simulink model "symmetric_lht"  (R2020a)
settings: Solver=FixedStepDiscrete  StartTime=0.0  StopTime=inf  RelTol=1e-3
values from neighbouring files (symbols this model uses):
  fs = fclk(1)*1e6    [setupSystem.m]
  height = heightName(nameIdx)    [setupSystem.m]
  inarray = uint8(simDirNew)    [setupSystem.m]
  nRho = maxRho*2    [setupSystem.m]
  nTheta = length(theta)    [setupSystem.m]
  theta = 0:1:179    [SymmetricLHT.m]    (also in setupSystem.m = (0:1:179))
  width = widthName(nameIdx)    [setupSystem.m]
undefined symbols (not defined in the file or in its folder): rhoBits, rhoMax
libraries: hdlsllib x35, simulink x25, dspsrcs4 x1
(part 2 of 2)

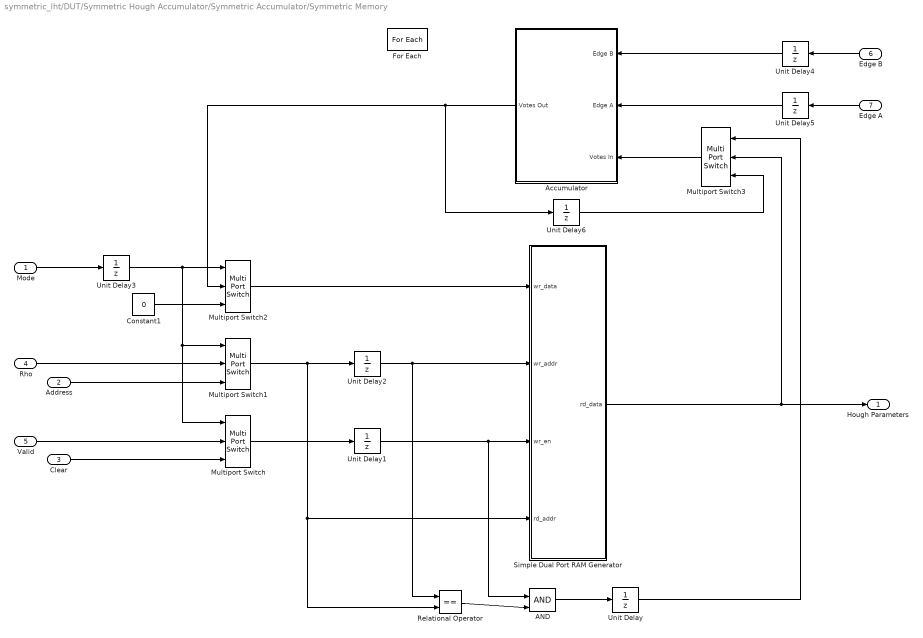
== system symmetric_lht/DUT/Symmetric Hough Accumulator/Symmetric Accumulator/Symmetric Memory ==
  Mode : Inport
  Address : Inport  Port=2
  Clear : Inport  Port=3
  Rho : Inport  Port=4  Partition=on  PartitionDimension=2  PartitionWidth=1  PartitionOffset=0
  Valid : Inport  Port=5
  Edge B : Inport  Port=6
  Edge A : Inport  Port=7
  AND : Logic  IconShape=distinctive  AllPortsSameDT=off  OutDataTypeStr=boolean
  Accumulator : Subsystem
  Constant1 : Constant  Value=0  OutDataTypeStr=fixdt(0,rhoBits*2,0)  SampleTime=-1
  For Each : ForEach  DisableCoverage=on
  Multiport Switch{,1..3} (4 alike) : MultiPortSwitch  DataPortOrder=Zero-based contiguous  Inputs=2  zeroidx=on
  Relational Operator : RelationalOperator  Operator===  OutDataTypeStr=boolean  RndMeth=Simplest
  Simple Dual Port RAM Generator : Subsystem  VariantControl=other_bits  mask{b=22, d=1470, b_hidden=22, d_hidden=1470}
      mask prompts: b "Data width:"; d "Depth:"
      mask init:
      | if d == d_hidden
      |     return
      | end
      | 
      | dBase = evalin('base', get_param(gcb, 'd'));
      | bBase = evalin('base', get_param(gcb, 'b'));
      | 
      | fprintf('HPS Memory updated...\r\n');
      | 
      | set_param(gcb, 'd_hidden', int2str(dBase));
      | set_param(gcb, 'b_hidden', int2str(bBase));
      | 
      | % Xilinx RAM Initialisation
      | xl_config = [512, 72;
      |             1024, 36;
      |             2048, 18;
      |             4096, 9;
      |             8192, 4;
      |             16384, 2;
      |             32768, 1];
      | 
      | % Get length of Xilinx Configuration
      | sizeram = size(xl_config);
      |         
      | % Get the RAM Configuration based on the data width
      | for i = 1:sizeram(1)
      |     if b <= xl_config(i, 2)
      |         a = xl_config(i, :);
      |     end
      | end
      | 
      | % Get number of BRAM required (including half BRAM)
      | numbram = ceil((d/a(1))/0.5)*0.5;
      | fullbram = floor(numbram); % Integer
      | halfbram = (numbram-floor(numbram)) ~= 0; % Boolean
      | 
      | % Get all blocks and delete everything excepts ports
      | H = get(find_system(gcb, 'FindAll', 'on', 'type', 'block'));
      | todelete = setdiff(strcat(repmat({[gcb '/']}, numel(H.Blocks), 1),  H.Blocks),...
      |     strcat(repmat({[gcb '/']}, 5, 1),...
      |     {'wr_data'; 'wr_addr'; 'wr_en'; 'rd_addr'; 'rd_data'}));
      | delete_block(todelete);
      | 
      | % Delete lines
      | for i = 1:numel(H.Lines)
      |     delete_line(H.Lines(i).Handle)
      | end
      | 
      | % Generate full BRAMs
      | y = 0;
      | 
      | % If there is only one ram then the write enable should be directly
      | % connected to the first ram write enable. Else, the write address must be sliced
      | % and the upper bound (over a(2)) compared to zero. This will indicate if
      | % the first ram is the one to be written/read from.
      | 
      | % Common to both implementations
      | % Write Address Slice
      | add_block('hdlsllib/Logic and Bit Operations/Bit Slice',...
      |         [gcb, '/wr_address'], 'Position',...
      |         [160 130 250 170]);
      | % Set bitslice parameters
      | set_param([gcb, '/wr_address'],...
      |     'lidx', int2str(log2(a(1))-1));
      | set_param([gcb, '/wr_address'],...
      |     'ridx', int2str(0));
      | 
      | % Read Address Slice
      | add_block('hdlsllib/Logic and Bit Operations/Bit Slice',...
      |         [gcb, '/rd_address'], 'Position',...
      |         [160 330 250 370]);
      | % Set bitslice parameters
      | set_param([gcb, '/rd_address'],...
      |     'lidx', int2str(log2(a(1))-1));
      | set_param([gcb, '/rd_address'],...
      |     'ridx', int2str(0));
      | 
      | if ceil(numbram) == 1
      |     
      |     i = 1;
      |     
      |     % Set bitslice parameters
      |     set_param([gcb, '/rd_address'],...
      |         'lidx', int2str(ceil(log2(d))-1));
      |     set_param([gcb, '/wr_address'],...
      |         'lidx', int2str(ceil(log2(d))-1));
      |     
      |     % Add Simple RAM
      |     add_block('hdlsllib/HDL RAMs/Simple Dual Port RAM',...
      |         [gcb, '/simple_ram_', int2str(i-1)], 'Position',...
      |         [635 0+600*y 635+200 400+600*y]);
      | 
      |     % Set RAM parameters
      |     set_param([gcb, '/simple_ram_', int2str(i-1)],...
      |         'ram_size', int2str(ceil(log2(d))));
      | 
      |     % Connect "wr_data" to "simple_ram_i"
      |     add_line(gcb, ['wr_data/1'], ['simple_ram_', int2str(i-1), '/1'],...
      |         'autorouting', 'on');
      |     
      |     % Connect "wr_addr" to "wr_address"
      |     add_line(gcb, ['wr_addr/1'], ['wr_address/1'],...
      |         'autorouting', 'on');
      | 
      |     % Connect "wr_address" to "simple_ram_i"
      |     add_line(gcb, ['wr_address/1'], ['simple_ram_', int2str(i-1), '/2'],...
      |         'autorouting', 'on');
      | 
      |     % Connect "wr_en" to "simple_ram_i"
      |     add_line(gcb, ['wr_en/1'], ['simple_ram_', int2str(i-1), '/3'],...
      |         'autorouting', 'on');
      |     
      |     % Connect "rd_addr" to "rd_address"
      |     add_line(gcb, ['rd_addr/1'], ['rd_address/1'],...
      |         'autorouting', 'on');
      | 
      |     % Connect "rd_address" to "simple_ram_i"
      |     add_line(gcb, ['rd_address/1'], ['simple_ram_', int2str(i-1), '/4'],...
      |         'autorouting', 'on');
      |     
      |     % Connect "simple_ram_i" to "rd_data"
      |     add_line(gcb, ['simple_ram_', int2str(i-1), '/1'], ['rd_data/1'],...
      |         'autorouting', 'on');
      | 
      | else
      |     
      |     % Multiport Switch
      |     add_block('hdlsllib/Signal Routing/Multiport Switch',...
      |         [gcb, '/multiport_switch'], 'Position',...
      |         [1340 146 1405 250]);
      |     % Set multiport switch parameters
      |     set_param([gcb, '/multiport_switch'],...
      |         'Inputs', int2str(ceil(numbram)));
      |     set_param([gcb, '/multiport_switch'],...
      |         'DataPortOrder', 'Zero-based contiguous');
      | 
      |     % Add Constant Zero
      |     add_block('hdlsllib/Sources/Constant',...
      |         [gcb, '/zero'], 'Position',...
      |         [425 -65 455 -35]);
      |     set_param([gcb, '/zero'],...
      |         'Value', int2str(0));
      |     set_param([gcb, '/zero'],...
      |         'OutDataTypeStr', ['fixdt(0, ', int2str(ceil(numbram)), ', 0)']);
      | 
      |     % Add Vector Concatenate
      |     add_block('hdlsllib/Signal Routing/Vector Concatenate',...
      |         [gcb, '/vector_concatenate'], 'Position',...
      |         [1015, -113, 1025, 38]);
      |     set_param([gcb, '/vector_concatenate'],...
      |         'NumInputs', int2str(ceil(numbram)));
      | 
      |     % Add Bitwise-OR
      |     add_block('hdlsllib/Logic and Bit Operations/Bitwise Operator',...
      |         [gcb, '/bitwise_or'], 'Position',...
      |         [1165, -54, 1205, -16]);
      |     set_param([gcb, '/bitwise_or'],...
      |         'logicop', 'OR');
      |     set_param([gcb, '/bitwise_or'],...
      |         'UseBitMask', 0);
      |     set_param([gcb, '/bitwise_or'],...
      |         'NumInputPorts', int2str(1));
      | 
      |     % Add delay for bram access
      |     add_block('hdlsllib/Discrete/Delay',...
      |         [gcb, '/delay'], 'Position',...
      |         [1248, 60, 1282, 95]);
      |     set_param([gcb, '/delay'],...
      |         'DelayLength', int2str(1));
      |     
      |     % Add bitslice
      |     add_block('hdlsllib/Logic and Bit Operations/Bit Slice',...
      |         [gcb, '/wr_bitslice'], 'Position',...
      |         [-65 180 25 220]);
      | 
      |     % Set bitslice parameters
      |     set_param([gcb, '/wr_bitslice'],...
      |         'lidx', int2str(ceil(log2(d)-1)));
      |     set_param([gcb, '/wr_bitslice'],...
      |         'ridx', int2str(log2(a(1))));
      |     
      |     % Add bitslice
      |     add_block('hdlsllib/Logic and Bit Operations/Bit Slice',...
      |         [gcb, '/rd_bitslice'], 'Position',...
      |         [-65 280 25 320]);
      | 
      |     % Set bitslice parameters
      |     set_param([gcb, '/rd_bitslice'],...
      |         'lidx', int2str(ceil(log2(d)-1)));
      |     set_param([gcb, '/rd_bitslice'],...
      |         'ridx', int2str(log2(a(1))));
      |     
      |     for i = 1:ceil(numbram)
      |         
      |         %%%%% Begin Adding Blocks %%%%%
      |         % Add Simple RAM
      |         add_block('hdlsllib/HDL RAMs/Simple Dual Port RAM',...
      |             [gcb, '/simple_ram_', int2str(i-1)], 'Position',...
      |             [635 0+600*y 635+200 400+600*y]);
      | 
      |         % Set RAM parameters
      |         set_param([gcb, '/simple_ram_', int2str(i-1)],...
      |             'ram_size', int2str(log2(a(1))));
      | 
      |         % Add compare to constant
      |         add_block('hdlsllib/Logic and Bit Operations/Compare To Constant',...
      |             [gcb, '/wr_cmp2const_', int2str(i-1)], 'Position',...
      |             [190 225+y*600 220 255+y*600]); 
      | 
      |         % Set compare to zero parameters
      |         set_param([gcb, '/wr_cmp2const_', int2str(i-1)],...
      |             'relop', '==');
      | 
      |         % Set compare to zero parameters
      |         set_param([gcb, '/wr_cmp2const_', int2str(i-1)],...
      |             'const', int2str(i-1));
      |         
      |         % Add compare to constant
      |         add_block('hdlsllib/Logic and Bit Operations/Compare To Constant',...
      |             [gcb, '/rd_cmp2const_', int2str(i-1)], 'Position',...
      |             [190 445+y*600 220 475+y*600]); 
      | 
      |         % Set compare to zero parameters
      |         set_param([gcb, '/rd_cmp2const_', int2str(i-1)],...
      |             'relop', '==');
      | 
      |         % Set compare to zero parameters
      |         set_param([gcb, '/rd_cmp2const_', int2str(i-1)],...
      |             'const', int2str(i-1));
      | 
      |         % Add and logic
      |         add_block('hdlsllib/Logic and Bit Operations/Logical Operator',...
      |             [gcb, '/and_', int2str(i-1)], 'Position',...
      |             [420 231+600*y 455 264+600*y]);
      | 
      |         % Set and logic parameters
      |         set_param([gcb, '/and_', int2str(i-1)],...
      |             'Operator', 'AND');
      | 
      |         % Add Switch
      |         add_block('hdlsllib/Signal Routing/Switch',...
      |             [gcb, '/switch_', int2str(i-1)], 'Position',...
      |             [685 -113+600*y 785 -37+600*y]);
      | 
      |         % Set switch parameters
      |         set_param([gcb, '/switch_', int2str(i-1)],...
      |             'Threshold', int2str(1));
      | 
      |         % Add Constant
      |         add_block('hdlsllib/Sources/Constant',...
      |             [gcb, '/constant_', int2str(i-1)], 'Position',...
      |             [425 -115+600*y 455 -85+600*y]);
      | 
      |         % Set Constant parameters
      |         set_param([gcb, '/constant_', int2str(i-1)],...
      |             'Value', int2str(i-1));
      |         set_param([gcb, '/constant_', int2str(i-1)],...
      |             'OutDataTypeStr', ['fixdt(0, ', int2str(ceil(numbram)), ', 0)']);   
      | 
      |         %%%%% Begin Wire Connections %%%%%        
      |         % Connect "wr_data" to "simple_ram_i"
      |         add_line(gcb, 'wr_data/1', ['simple_ram_', int2str(i-1), '/1'],...
      |             'autorouting','on');
      | 
      |         % Connect "wr_address" to "simple_ram_i"
      |         add_line(gcb, 'wr_address/1', ['simple_ram_', int2str(i-1), '/2'],...
      |             'autorouting','on');
      | 
      |         % Connect "rd_address" to "simple_ram_i"
      |         add_line(gcb, 'rd_address/1', ['simple_ram_', int2str(i-1), '/4'],...
      |             'autorouting','on');
      | 
      |         % Connect "constant_i" to "switch_i"
      |         add_line(gcb, ['constant_', int2str(i-1), '/1'], ['switch_', int2str(i-1), '/1'],...
      |             'autorouting','on');
      | 
      |         % Connect "zero" to "switch_i"
      |         add_line(gcb, 'zero/1', ['switch_', int2str(i-1), '/3'],...
      |             'autorouting','on');
      | 
      |         % Connect "switch_i" to "vector_concatenate"
      |         add_line(gcb, ['switch_', int2str(i-1), '/1'], ['vector_concatenate/', int2str(i)],...
      |             'autorouting','on');
      | 
      |         % Connect "rd_address" to "simple_ram_i"
      |         add_line(gcb, ['simple_ram_', int2str(i-1), '/1'], ['multiport_switch/', int2str(i+1)],...
      |             'autorouting','on');
      | 
      |         % Connect "bitslice_i" to "wr_cmp2const_i"
      |         add_line(gcb, ['wr_bitslice/1'], ['wr_cmp2const_', int2str(i-1), '/1'],...
      |             'autorouting','on');
      |         
      |         % Connect "bitslice_i" to "rd_cmp2const_i"
      |         add_line(gcb, ['rd_bitslice/1'], ['rd_cmp2const_', int2str(i-1), '/1'],...
      |             'autorouting','on');
      | 
      |         % Connect "wr_en" to "and_i"
      |         add_line(gcb, ['wr_en/1'], ['and_', int2str(i-1), '/2'],...
      |             'autorouting','on');
      | 
      |         % Connect "and_i" to "simple_ram_0"
      |         add_line(gcb, ['and_', int2str(i-1), '/1'], ['simple_ram_', int2str(i-1), '/3'],...
      |             'autorouting','on');
      | 
      |         % Connect "wr_cmp2const_i" to "and_i"
      |         add_line(gcb, ['wr_cmp2const_', int2str(i-1), '/1'], ['and_', int2str(i-1), '/1'],...
      |             'autorouting','on');
      | 
      |         % Connect "rd_cmp2const_i" to "switch_i"
      |         add_line(gcb, ['rd_cmp2const_', int2str(i-1), '/1'], ['switch_', int2str(i-1), '/2'],...
      |             'autorouting','on');
      |          
      |         % Update coordinates
      |         y = y + 1;
      |         
      |     end
      |     
      |     % Connect "rd_addr" to "bitslice_i"
      |     add_line(gcb, ['rd_addr/1'], ['rd_bitslice/1'],...
      |         'autorouting','on');
      |     
      |     % Connect "wr_addr" to "bitslice_i"
      |     add_line(gcb, ['wr_addr/1'], ['wr_bitslice/1'],...
      |         'autorouting','on');
      |     
      |     % Connect "wr_addr" to "wr_address"
      |     add_line(gcb, 'wr_addr/1', ['wr_address', '/1'],...
      |         'autorouting','on');
      | 
      |     % Connect "rd_addr" to "rd_address"
      |     add_line(gcb, 'rd_addr/1', ['rd_address', '/1'],...
      |         'autorouting','on');
      | 
      |     % Connect "vector_concatenate" to "bitwise_or"
      |     add_line(gcb, ['vector_concatenate/1'], ['bitwise_or/1'],...
      |         'autorouting','on');
      | 
      |     % Connect "bitwise_or" to "delay"
      |     add_line(gcb, ['bitwise_or/1'], ['delay/1'],...
      |         'autorouting','on');
      | 
      |     % Connect "delay" to "multiport_switch"
      |     add_line(gcb, ['delay/1'], ['multiport_switch/1'],...
      |         'autorouting','on');
      | 
      |     % Connect "multiport_switch" to "rd_data"
      |     add_line(gcb, ['multiport_switch/1'], ['rd_data/1'],...
      |         'autorouting','on');
      |     
      | end
      | 
      | % If there is a half bram we must change a few parameters. Firstly, delete
      | % the write and read address lines. Then add bitslice blocks to reduce the
      | % address space in half. Connect rd_addr and wr_addr to the corresponding ports
      | % on the bram. Finally, change the address depth.
      | if halfbram
      |     
      |     if ceil(numbram) > 1
      |         
      |         % Delete lines
      |         delete_line(gcb, ['wr_address/1'], ['simple_ram_', int2str(i-1), '/2'])
      |         delete_line(gcb, ['rd_address/1'], ['simple_ram_', int2str(i-1), '/4'])
      |         
      |         % Write Address half ram Slice
      |         add_block('hdlsllib/Logic and Bit Operations/Bit Slice',...
      |                 [gcb, '/wr_address_hr'], 'Position',...
      |                 [160 130+(y-1)*600 250 170+(y-1)*600]);
      |         % Set bitslice parameters
      |         set_param([gcb, '/wr_address_hr'],...
      |             'lidx', int2str(log2(a(1))-2));
      |         set_param([gcb, '/wr_address_hr'],...
      |             'ridx', int2str(0));
      | 
      |         % Read Address half ram Slice
      |         add_block('hdlsllib/Logic and Bit Operations/Bit Slice',...
      |                 [gcb, '/rd_address_hr'], 'Position',...
      |                 [160 330+(y-1)*600 250 370+(y-1)*600]);
      |         % Set bitslice parameters
      |         set_param([gcb, '/rd_address_hr'],...
      |             'lidx', int2str(log2(a(1))-2));
      |         set_param([gcb, '/rd_address_hr'],...
      |             'ridx', int2str(0));
      | 
      |         % Connect "wr_addr" to "wr_address_hr"
      |         add_line(gcb, 'wr_addr/1', ['wr_address_hr', '/1'],...
      |             'autorouting','on');
      | 
      |         % Connect "rd_addr" to "rd_address_hr"
      |         add_line(gcb, 'rd_addr/1', ['rd_address_hr', '/1'],...
      |             'autorouting','on');
      | 
      |         % Connect "wr_address_hr" to "simple_ram_i"
      |         add_line(gcb, ['wr_address_hr', '/1'], ['simple_ram_', int2str(i-1), '/2'],...
      |             'autorouting','on');
      | 
      |         % Connect "rd_address_hr" to "simple_ram_i"
      |         add_line(gcb, ['rd_address_hr', '/1'], ['simple_ram_', int2str(i-1), '/4'],...
      |             'autorouting','on');
      |         
      |         % Update the ram parameters (address bits)
      |         set_param([gcb, '/simple_ram_', int2str(i-1)],...
      |             'ram_size', int2str(log2(a(1)/2)));
      | 
      |     else
      |         % Set bitslice parameters
      |         % set_param([gcb, '/wr_address'],...
      |         %     'lidx', int2str(log2(a(1))-2));
      |         % set_param([gcb, '/wr_address'],...
      |         %     'ridx', int2str(0));
      |         % Set bitslice parameters
      |         % set_param([gcb, '/rd_address'],...
      |         %     'lidx', int2str(log2(a(1))-2));
      |         % set_param([gcb, '/rd_address'],...
      |         %     'ridx', int2str(0));
      |         
      |     end
      |     
      | 
      |     
      | end
  Unit Delay{,1..6} (7 alike) : UnitDelay  SampleTime=-1  HasFrameUpgradeWarning=on
  Hough Parameters : Outport  ConcatenationDimension=2
  wires:
  Unit Delay/1 -> Multiport Switch3/1
  Unit Delay6/1 -> Multiport Switch3/3
  Multiport Switch3/1 -> Accumulator/3(Votes In)
  AND/1 -> Unit Delay/1
  Relational Operator/1 -> AND/2
  Valid/1 -> Multiport Switch/2
  Simple Dual Port RAM Generator/1(rd_data) -> Multiport Switch3/2, Hough Parameters/1
  Unit Delay5/1 -> Accumulator/2(Edge A)
  Unit Delay4/1 -> Accumulator/1(Edge B)
  Constant1/1 -> Multiport Switch2/3
  Unit Delay2/1 -> Simple Dual Port RAM Generator/2(wr_addr), Relational Operator/1
  Unit Delay1/1 -> Simple Dual Port RAM Generator/3(wr_en), AND/1
  Rho/1 -> Multiport Switch1/2
  Clear/1 -> Multiport Switch/3
  Unit Delay3/1 -> Multiport Switch/1, Multiport Switch1/1, Multiport Switch2/1
  Multiport Switch2/1 -> Simple Dual Port RAM Generator/1(wr_data)
  Multiport Switch/1 -> Unit Delay1/1
  Mode/1 -> Unit Delay3/1
  Edge B/1 -> Unit Delay4/1
  Address/1 -> Multiport Switch1/3
  Edge A/1 -> Unit Delay5/1
  Multiport Switch1/1 -> Simple Dual Port RAM Generator/4(rd_addr), Relational Operator/2, Unit Delay2/1
  Accumulator/1(Votes Out) -> Multiport Switch2/2, Unit Delay6/1

== system symmetric_lht/DUT/Symmetric Hough Kernel/FIFO Half Rate System/FIFO Half Rate A ==
  In : Inport
  Push : Inport  Port=2
  Delay : Delay  DelayLength=1
  HDL FIFO : hdlsllib/HDL RAMs/HDL FIFO  fifo_size=(width/2)/2+1  mode=Classic  ratio=2  push_msg=Error  pop_msg=Error  show_empty=on  show_full=off  show_num=off  LabelModeActiveChoice_Mode=Classic
      settings: SourceProductBaseCode=SL
  NOT : Logic  Operator=NOT  IconShape=distinctive  AllPortsSameDT=off  OutDataTypeStr=boolean
  Rate Transition : RateTransition
  Out : Outport
  Valid : Outport  Port=2
  wires:
  HDL FIFO/2 -> Rate Transition/1
  Push/1 -> HDL FIFO/2
  In/1 -> HDL FIFO/1
  HDL FIFO/1 -> Out/1
  Rate Transition/1 -> NOT/1
  NOT/1 -> HDL FIFO/3, Delay/1
  Delay/1 -> Valid/1

== system symmetric_lht/DUT/Symmetric Hough Kernel/FIFO Half Rate System/FIFO Half Rate B ==
  In : Inport
  Push : Inport  Port=2
  Delay : Delay  DelayLength=1
  HDL FIFO : hdlsllib/HDL RAMs/HDL FIFO  fifo_size=(width/2)/2+1  mode=Classic  ratio=2  push_msg=Error  pop_msg=Error  show_empty=on  show_full=off  show_num=off  LabelModeActiveChoice_Mode=Classic
      settings: SourceProductBaseCode=SL
  NOT : Logic  Operator=NOT  IconShape=distinctive  AllPortsSameDT=off  OutDataTypeStr=boolean
  Rate Transition : RateTransition
  Out : Outport
  Valid : Outport  Port=2
  wires:
  Delay/1 -> Valid/1
  NOT/1 -> Delay/1, HDL FIFO/3
  Rate Transition/1 -> NOT/1
  HDL FIFO/1 -> Out/1
  In/1 -> HDL FIFO/1
  Push/1 -> HDL FIFO/2
  HDL FIFO/2 -> Rate Transition/1

== system symmetric_lht/DUT/Symmetric Hough Kernel/Symmetric Kernel/Coordinate Counters ==
  valid : Inport
  AND : Logic  IconShape=distinctive  AllPortsSameDT=off  OutDataTypeStr=boolean
  Compare To Constant : simulink/Logic and Bit Operations/Compare To Constant  relop===  const=width/2  OutDataTypeStr=boolean
  Compare To Zero : simulink/Logic and Bit Operations/Compare To Zero  relop=>=  OutDataTypeStr=boolean
  Compare To Zero1 : simulink/Logic and Bit Operations/Compare To Zero  relop=>=  OutDataTypeStr=boolean
  Counter : hdlsllib/Sources/HDL Counter  CountType=Count limited  CountInit=-height/2  CountStep=1  CountMax=height/2-1  CountFromType=Initial value  CountFrom=-height/2  CountResetPort=off  CountLoadPort=off  CountEnbPort=on  CountDirPort=off  CountDataType=Signed  CountWordLen=ceil(log2(height+1))  CountFracLen=0  CountSampTime=1
  Increment Real World : simulink/Additional Math & Discrete/Additional Math: Increment - Decrement/Increment Real World
      settings: SourceProductBaseCode=SL
  Increment Real World1 : simulink/Additional Math & Discrete/Additional Math: Increment - Decrement/Increment Real World
      settings: SourceProductBaseCode=SL
  Multiport Switch : MultiPortSwitch  DataPortOrder=Zero-based contiguous  Inputs=2  zeroidx=on
  Multiport Switch1 : MultiPortSwitch  DataPortOrder=Zero-based contiguous  Inputs=2  zeroidx=on
  X Counter : hdlsllib/Sources/HDL Counter  CountType=Count limited  CountInit=1  CountStep=1  CountMax=width/2  CountFromType=Initial value  CountFrom=1  CountResetPort=off  CountLoadPort=off  CountEnbPort=on  CountDirPort=off  CountDataType=Unsigned  CountWordLen=ceil(log2(width/2+1))  CountFracLen=0  CountSampTime=1
  x : Outport  VectorParamsAs1DForOutWhenUnconnected=off
  y : Outport  Port=2  VectorParamsAs1DForOutWhenUnconnected=off
  yp1 : Outport  Port=3  VectorParamsAs1DForOutWhenUnconnected=off
  y relative : Outport  Port=4  VectorParamsAs1DForOutWhenUnconnected=off
  wires:
  valid/1 -> AND/2, X Counter/1
  X Counter/1 -> x/1, Compare To Constant/1
  AND/1 -> Counter/1
  Compare To Constant/1 -> AND/1
  Multiport Switch/1 -> y/1
  Counter/1 -> Multiport Switch/2, y relative/1, Increment Real World/1, Compare To Zero/1
  Compare To Zero/1 -> Multiport Switch/1
  Increment Real World1/1 -> Multiport Switch1/3
  Compare To Zero1/1 -> Multiport Switch1/1
  Increment Real World/1 -> Increment Real World1/1, Multiport Switch1/2, Compare To Zero1/1, Multiport Switch/3
  Multiport Switch1/1 -> yp1/1

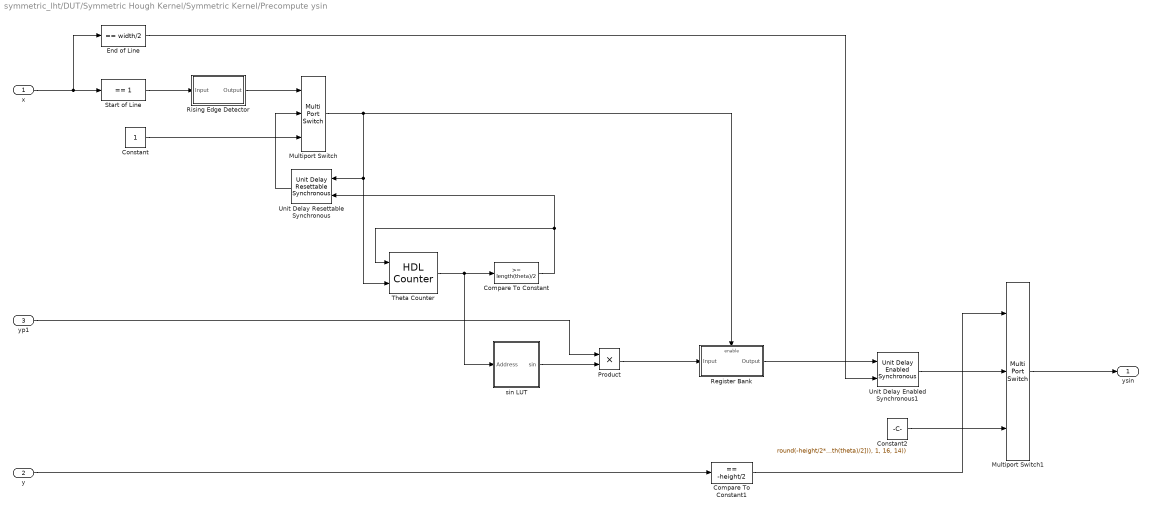
== system symmetric_lht/DUT/Symmetric Hough Kernel/Symmetric Kernel/Precompute ysin ==
  x : Inport
  y : Inport  Port=2
  yp1 : Inport  Port=3
  Compare To Constant : simulink/Logic and Bit Operations/Compare To Constant  relop=>=  const=length(theta)/2  OutDataTypeStr=boolean
  Compare To Constant1 : simulink/Logic and Bit Operations/Compare To Constant  relop===  const=-height/2  OutDataTypeStr=boolean
  Constant : Constant  OutDataTypeStr=boolean  SampleTime=-1
  Constant2 : Constant  Value=round(-height/2*fi(sin(deg2rad([0:1:length(theta)/2])), 1, 16, 14))  OutDataTypeStr=fixdt(1,ceil(log2(height+1)),0)  SampleTime=-1
  End of Line : simulink/Logic and Bit Operations/Compare To Constant  relop===  const=width/2  OutDataTypeStr=boolean
  Multiport Switch : MultiPortSwitch  DataPortOrder=Zero-based contiguous  Inputs=2  zeroidx=on
  Multiport Switch1 : MultiPortSwitch  DataPortOrder=Zero-based contiguous  Inputs=2  zeroidx=on
  Product : Product  RndMeth=Round  SaturateOnIntegerOverflow=on  OutDataTypeStr=Inherit: Same as first input
  Register Bank : Subsystem
  Rising Edge Detector : Subsystem
  Start of Line : simulink/Logic and Bit Operations/Compare To Constant  relop===  const=1  OutDataTypeStr=boolean
  Theta Counter : hdlsllib/Sources/HDL Counter  CountType=Count limited  CountInit=0  CountStep=1  CountMax=length(theta)/2  CountFromType=Initial value  CountFrom=0  CountResetPort=on  CountLoadPort=off  CountEnbPort=on  CountDirPort=off  CountDataType=Unsigned  CountWordLen=ceil(log2(length(theta)))  CountFracLen=0  CountSampTime=1
  Unit Delay Enabled Synchronous1 : hdlsllib/Discrete/Unit Delay Enabled Synchronous  InitialCondition=0.0  SampleTime=-1
      settings: SourceProductBaseCode=SL
  Unit Delay Resettable Synchronous : hdlsllib/Discrete/Unit Delay Resettable Synchronous  InitialCondition=0.0  SampleTime=-1
      settings: SourceProductBaseCode=SL
  sin LUT : Subsystem
  ysin : Outport  VectorParamsAs1DForOutWhenUnconnected=off
  wires:
  x/1 -> End of Line/1, Start of Line/1
  Start of Line/1 -> Rising Edge Detector/1(Input)
  Multiport Switch/1 -> Register Bank/Enable, Unit Delay Resettable Synchronous/1, Theta Counter/2
  Unit Delay Resettable Synchronous/1 -> Multiport Switch/2
  Constant/1 -> Multiport Switch/3
  Theta Counter/1 -> sin LUT/1(Address), Compare To Constant/1
  Rising Edge Detector/1(Output) -> Multiport Switch/1
  Multiport Switch1/1 -> ysin/1
  Constant2/1 -> Multiport Switch1/3
  Compare To Constant1/1 -> Multiport Switch1/1
  Product/1 -> Register Bank/1(Input)
  y/1 -> Compare To Constant1/1
  Compare To Constant/1 -> Unit Delay Resettable Synchronous/2, Theta Counter/1
  Unit Delay Enabled Synchronous1/1 -> Multiport Switch1/2
  End of Line/1 -> Unit Delay Enabled Synchronous1/2
  Register Bank/1(Output) -> Unit Delay Enabled Synchronous1/1
  yp1/1 -> Product/1
  sin LUT/1(sin) -> Product/2

== system symmetric_lht/DUT/Symmetric Hough Kernel/Symmetric Kernel/Quadrant Control ==
  Valid : Inport
  Delay : Delay  DelayLength=1  ShowEnablePort=on
      settings: InputPortMap=u0,e6
  First Quadrant Valid : Logic  IconShape=distinctive  AllPortsSameDT=off  OutDataTypeStr=boolean
  NOT : Logic  Operator=NOT  IconShape=distinctive  AllPortsSameDT=off  OutDataTypeStr=boolean
  Second Quadrant Valid : Logic  IconShape=distinctive  AllPortsSameDT=off  OutDataTypeStr=boolean
  Q1 Valid : Outport
  Q2 Valid : Outport  Port=2
  Q Selector : Outport  Port=3
  wires:
  Second Quadrant Valid/1 -> Q2 Valid/1
  First Quadrant Valid/1 -> Q1 Valid/1
  Delay/1 -> Q Selector/1, NOT/1, Second Quadrant Valid/2
  NOT/1 -> Delay/1, First Quadrant Valid/2
  Valid/1 -> Delay/2, Second Quadrant Valid/1, First Quadrant Valid/1

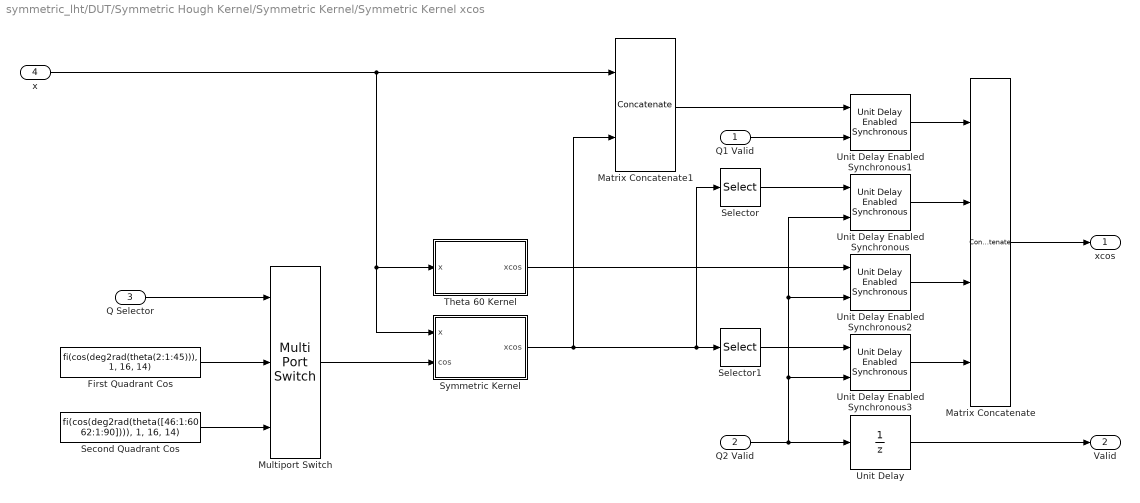
== system symmetric_lht/DUT/Symmetric Hough Kernel/Symmetric Kernel/Symmetric Kernel xcos ==
  Q1 Valid : Inport
  Q2 Valid : Inport  Port=2
  Q Selector : Inport  Port=3
  x : Inport  Port=4
  First Quadrant Cos : Constant  Value=fi(cos(deg2rad(theta(2:1:45))), 1, 16, 14)  VectorParams1D=off  OutDataTypeStr=fixdt(1,16,14)  SampleTime=-1
  Matrix Concatenate : Concatenate  NumInputs=4  Mode=Multidimensional array  ConcatenateDimension=2
  Matrix Concatenate1 : Concatenate  Mode=Multidimensional array  ConcatenateDimension=2
  Multiport Switch : MultiPortSwitch  DataPortOrder=Zero-based contiguous  Inputs=2  zeroidx=on
  Second Quadrant Cos : Constant  Value=fi(cos(deg2rad(theta([46:1:60 62:1:90]))), 1, 16, 14)  VectorParams1D=off  OutDataTypeStr=fixdt(1,16,14)  SampleTime=-1
  Selector : Selector  InputPortWidth=44  IndexOptions=Index vector (dialog)  Indices=[1:1:15]  OutputSizes=1
  Selector1 : Selector  InputPortWidth=44  IndexOptions=Index vector (dialog)  Indices=[16:1:44]  OutputSizes=1
  Symmetric Kernel : Subsystem  VariantControl=dsp48e
  Theta 60 Kernel : Subsystem
  Unit Delay : UnitDelay  SampleTime=-1  HasFrameUpgradeWarning=on
  Unit Delay Enabled Synchronous{,1..3} (4 alike) : hdlsllib/Discrete/Unit Delay Enabled Synchronous  InitialCondition=0.0  SampleTime=-1
      settings: SourceProductBaseCode=SL
  xcos : Outport
  Valid : Outport  Port=2
  wires:
  Q1 Valid/1 -> Unit Delay Enabled Synchronous1/2
  First Quadrant Cos/1 -> Multiport Switch/2
  Unit Delay Enabled Synchronous1/1 -> Matrix Concatenate/1
  Second Quadrant Cos/1 -> Multiport Switch/3
  Q Selector/1 -> Multiport Switch/1
  Unit Delay Enabled Synchronous/1 -> Matrix Concatenate/2
  Q2 Valid/1 -> Unit Delay/1, Unit Delay Enabled Synchronous3/2, Unit Delay Enabled Synchronous2/2, Unit Delay Enabled Synchronous/2
  Matrix Concatenate/1 -> xcos/1
  Unit Delay/1 -> Valid/1
  x/1 -> Symmetric Kernel/1(x), Theta 60 Kernel/1(x), Matrix Concatenate1/1
  Multiport Switch/1 -> Symmetric Kernel/2(cos)
  Matrix Concatenate1/1 -> Unit Delay Enabled Synchronous1/1
  Symmetric Kernel/1(xcos) -> Matrix Concatenate1/2, Selector1/1, Selector/1
  Unit Delay Enabled Synchronous2/1 -> Matrix Concatenate/3
  Unit Delay Enabled Synchronous3/1 -> Matrix Concatenate/4
  Selector/1 -> Unit Delay Enabled Synchronous/1
  Selector1/1 -> Unit Delay Enabled Synchronous3/1
  Theta 60 Kernel/1(xcos) -> Unit Delay Enabled Synchronous2/1

== system symmetric_lht/DUT/Symmetric Hough Accumulator/Symmetric Accumulator/Symmetric Memory/Accumulator ==
  Edge B : Inport
  Edge A : Inport  Port=2
  Votes In : Inport  Port=3
  Add1 : Sum  OutDataTypeStr=Inherit: Same as first input
  Add2 : Sum  OutDataTypeStr=Inherit: Same as first input
  Bit Concat : hdlsllib/Logic and Bit Operations/Bit Concat  numInputs=2
  Bit Slice2 : hdlsllib/Logic and Bit Operations/Bit Slice  lidx=rhoBits*2-1  ridx=rhoBits
      settings: SourceProductBaseCode=SL
  Bit Slice4 : hdlsllib/Logic and Bit Operations/Bit Slice  lidx=rhoBits-1  ridx=0
      settings: SourceProductBaseCode=SL
  Votes Out : Outport
  wires:
  Edge A/1 -> Add2/2
  Bit Slice4/1 -> Add2/1
  Edge B/1 -> Add1/2
  Bit Slice2/1 -> Add1/1
  Add2/1 -> Bit Concat/2
  Bit Concat/1 -> Votes Out/1
  Votes In/1 -> Bit Slice2/1, Bit Slice4/1
  Add1/1 -> Bit Concat/1

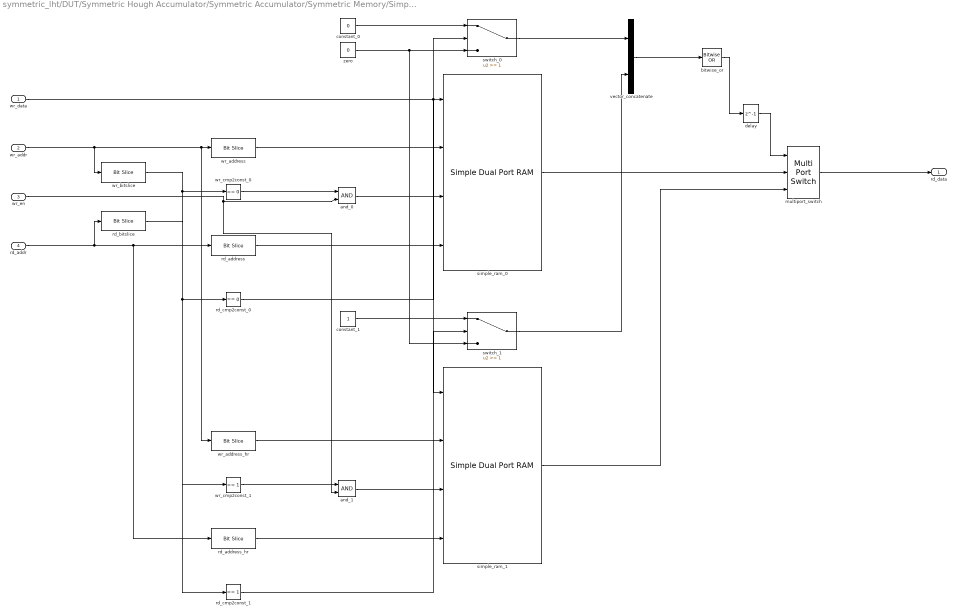
== system symmetric_lht/DUT/Symmetric Hough Accumulator/Symmetric Accumulator/Symmetric Memory/Simple Dual Port RAM Generator ==
  wr_data : Inport
  wr_addr : Inport  Port=2
  wr_en : Inport  Port=3
  rd_addr : Inport  Port=4
  and_0 : Logic  AllPortsSameDT=off  OutDataTypeStr=boolean
  and_1 : Logic  AllPortsSameDT=off  OutDataTypeStr=boolean
  bitwise_or : simulink/Logic and Bit Operations/Bitwise Operator  logicop=OR  UseBitMask=off  BitMask=bin2dec('11011001')  BitMaskRealWorld=Stored Integer
  constant_0 : Constant  Value=0  OutDataTypeStr=fixdt(0, 2, 0)  SampleTime=-1
  constant_1 : Constant  OutDataTypeStr=fixdt(0, 2, 0)  SampleTime=-1
  delay : Delay  DelayLength=1
  multiport_switch : MultiPortSwitch  DataPortOrder=Zero-based contiguous  Inputs=2  zeroidx=on
  rd_address : hdlsllib/Logic and Bit Operations/Bit Slice  lidx=9  ridx=0
      settings: SourceProductBaseCode=SL
  rd_address_hr : hdlsllib/Logic and Bit Operations/Bit Slice  lidx=8  ridx=0
      settings: SourceProductBaseCode=SL
  rd_bitslice : hdlsllib/Logic and Bit Operations/Bit Slice  lidx=10  ridx=10
      settings: SourceProductBaseCode=SL
  rd_cmp2const_0 : simulink/Logic and Bit Operations/Compare To Constant  relop===  const=0  OutDataTypeStr=boolean
  rd_cmp2const_1 : simulink/Logic and Bit Operations/Compare To Constant  relop===  const=1  OutDataTypeStr=boolean
  simple_ram_0 : hdlsllib/HDL RAMs/Simple Dual Port RAM  ram_size=10
      settings: SourceProductBaseCode=SL
  simple_ram_1 : hdlsllib/HDL RAMs/Simple Dual Port RAM  ram_size=9
      settings: SourceProductBaseCode=SL
  switch_0 : Switch  Threshold=1
  switch_1 : Switch  Threshold=1
  vector_concatenate : Concatenate
  wr_address : hdlsllib/Logic and Bit Operations/Bit Slice  lidx=9  ridx=0
      settings: SourceProductBaseCode=SL
  wr_address_hr : hdlsllib/Logic and Bit Operations/Bit Slice  lidx=8  ridx=0
      settings: SourceProductBaseCode=SL
  wr_bitslice : hdlsllib/Logic and Bit Operations/Bit Slice  lidx=10  ridx=10
      settings: SourceProductBaseCode=SL
  wr_cmp2const_0 : simulink/Logic and Bit Operations/Compare To Constant  relop===  const=0  OutDataTypeStr=boolean
  wr_cmp2const_1 : simulink/Logic and Bit Operations/Compare To Constant  relop===  const=1  OutDataTypeStr=boolean
  zero : Constant  Value=0  OutDataTypeStr=fixdt(0, 2, 0)  SampleTime=-1
  rd_data : Outport
  wires:
  wr_data/1 -> simple_ram_0/1, simple_ram_1/1
  wr_address/1 -> simple_ram_0/2
  rd_address/1 -> simple_ram_0/4
  constant_0/1 -> switch_0/1
  zero/1 -> switch_0/3, switch_1/3
  switch_0/1 -> vector_concatenate/1
  simple_ram_0/1 -> multiport_switch/2
  wr_bitslice/1 -> wr_cmp2const_0/1, wr_cmp2const_1/1
  rd_bitslice/1 -> rd_cmp2const_0/1, rd_cmp2const_1/1
  wr_en/1 -> and_0/2, and_1/2
  and_0/1 -> simple_ram_0/3
  wr_cmp2const_0/1 -> and_0/1
  rd_cmp2const_0/1 -> switch_0/2
  constant_1/1 -> switch_1/1
  switch_1/1 -> vector_concatenate/2
  simple_ram_1/1 -> multiport_switch/3
  and_1/1 -> simple_ram_1/3
  wr_cmp2const_1/1 -> and_1/1
  rd_cmp2const_1/1 -> switch_1/2
  rd_addr/1 -> rd_address/1, rd_address_hr/1, rd_bitslice/1
  wr_addr/1 -> wr_address/1, wr_address_hr/1, wr_bitslice/1
  vector_concatenate/1 -> bitwise_or/1
  bitwise_or/1 -> delay/1
  delay/1 -> multiport_switch/1
  multiport_switch/1 -> rd_data/1
  wr_address_hr/1 -> simple_ram_1/2
  rd_address_hr/1 -> simple_ram_1/4

== system symmetric_lht/DUT/Symmetric Hough Kernel/Symmetric Kernel/Precompute ysin/Register Bank ==
  Input : Inport
  Enable : EnablePort
  Tapped Delay : simulink/Discrete/Tapped Delay  vinit=0  samptime=-1  NumDelays=length(theta)/2  DelayOrder=Oldest  includeCurrent=on
  Output : Outport  InitialOutput=0  VectorParamsAs1DForOutWhenUnconnected=off
  wires:
  Tapped Delay/1 -> Output/1
  Input/1 -> Tapped Delay/1

== system symmetric_lht/DUT/Symmetric Hough Kernel/Symmetric Kernel/Precompute ysin/Rising Edge Detector ==
  Input : Inport
  AND : Logic  IconShape=distinctive  AllPortsSameDT=off  OutDataTypeStr=boolean
  Delay : Delay  DelayLength=1
  NOT : Logic  Operator=NOT  IconShape=distinctive  AllPortsSameDT=off  OutDataTypeStr=boolean
  Output : Outport  VectorParamsAs1DForOutWhenUnconnected=off
  wires:
  AND/1 -> Output/1
  Input/1 -> AND/2, Delay/1
  Delay/1 -> NOT/1
  NOT/1 -> AND/1

== system symmetric_lht/DUT/Symmetric Hough Kernel/Symmetric Kernel/Precompute ysin/sin LUT ==
  Address : Inport
  1-D Lookup Table : Lookup_n-D  NumberOfTableDimensions=1  BreakpointsForDimension1=[0:1:length(theta)/2]  IndexSearchMethod=Evenly spaced points  Table=fi(sin(deg2rad(theta(1:1:length(theta)/2+1))), 1, 16, 14)  InterpMethod=Flat  ExtrapMethod=Clip  DiagnosticForOutOfRangeInput=Error  InternalRulePriority=Speed  OutDataTypeStr=fixdt(1,16,14)  RndMeth=Simplest  InputSameDT=on
  sin : Outport
  wires:
  1-D Lookup Table/1 -> sin/1
  Address/1 -> 1-D Lookup Table/1

== system symmetric_lht/DUT/Symmetric Hough Kernel/Symmetric Kernel/Symmetric Kernel xcos/Symmetric Kernel ==
  x : Inport
  cos : Inport  Port=2
  Product : Product  RndMeth=Round  SaturateOnIntegerOverflow=on  OutDataTypeStr=Inherit: Same as first input
  xcos : Outport
  wires:
  x/1 -> Product/1
  cos/1 -> Product/2
  Product/1 -> xcos/1

== system symmetric_lht/DUT/Symmetric Hough Kernel/Symmetric Kernel/Symmetric Kernel xcos/Theta 60 Kernel ==
  x : Inport
  Bit Shift : hdlsllib/Logic and Bit Operations/Bit Shift  mode=Shift Right Logical  N=1
  Data Type Conversion : DataTypeConversion  OutDataTypeStr=fixdt(0,ceil(log2(width/2+1))+1,1)
  Data Type Conversion1 : DataTypeConversion  OutDataTypeStr=fixdt(0,ceil(log2(width/2+1)),0)  RndMeth=Round
  xcos : Outport
  wires:
  x/1 -> Data Type Conversion/1
  Data Type Conversion/1 -> Bit Shift/1
  Bit Shift/1 -> Data Type Conversion1/1
  Data Type Conversion1/1 -> xcos/1

== matlab function symmetric_lht/DUT/Symmetric Hough Accumulator/Accumulator Control/Accumulator FSM ==
  data: sofIn input; sofOut output; eofIn input; eofOut output; validOut output; phaseOut output; thetaOut output; modeOut output; addrOut output; voteOut output; clearOut output; thetaMax input; rhoMax input; stateDebug output
function [sofOut, eofOut, validOut, phaseOut, thetaOut, modeOut, addrOut, voteOut, clearOut, stateDebug] = AccumulatorControl(sofIn, eofIn, thetaMax, rhoMax)

IDLE = fi(0, 0, 3, 0);
VOTE = fi(1, 0, 3, 0);
READ_1 = fi(2, 0, 3, 0);
READ_2 = fi(3, 0, 3, 0);
CLEAR = fi(4, 0, 3, 0);

persistent current_state;
persistent theta_counter;
persistent address_counter;

if isempty(current_state)
    current_state = IDLE;
end

if isempty(theta_counter)
    theta_counter = fi(0, 0, 8, 0);
end

if isempty(address_counter)
    address_counter = fi(0, 0, 16, 0);
end

switch current_state
    case IDLE
        sofOut = false;
        eofOut = false; 
        validOut = false;
        modeOut = false;
        clearOut = false;
        phaseOut = false;
        thetaOut = theta_counter;
        addrOut = address_counter;
        stateDebug = current_state;
        
        if sofIn
            voteOut = true;
            current_state = VOTE;
        else
            voteOut = false;
        end
        
    case VOTE
        sofOut = false;
        eofOut = false; 
        validOut = false;
        modeOut = false;
        voteOut = true;
        clearOut = false;
        phaseOut = false;
        thetaOut = theta_counter;
        addrOut = address_counter;
        stateDebug = current_state;
        
        if eofIn
            current_state = READ_1;
        end
        
    case READ_1
        if theta_counter <= fi(0, 0, 8, 0) && ...
                address_counter <= fi(0, 0, 16, 0)
            sofOut = true;
        else
            sofOut = false;
        end
        
        eofOut = false;
        validOut = true;
        modeOut = true;
        voteOut = false;
        clearOut = false;
        phaseOut = false;
        thetaOut = theta_counter;
        addrOut = address_counter;
        stateDebug = current_state;
        
        if theta_counter >= thetaMax && address_counter >= rhoMax
            address_counter = fi(0, 0, 16, 0);
            theta_counter = fi(0, 0, 8, 0);
            current_state = READ_2;
        elseif address_counter >= rhoMax
            address_counter = fi(0, 0, 16, 0);
            theta_counter = fi(theta_counter + 1, 0, 8, 0);
        else
            address_counter = fi(address_counter + 1, 0, 16, 0);
        end
            
   case READ_2
        if theta_counter >= thetaMax && address_counter >= rhoMax
            eofOut = true;
        else
            eofOut = false;
        end
        
        sofOut = false;
        validOut = true;
        modeOut = true;
        voteOut = false;
        clearOut = false;
        phaseOut = true;
        thetaOut = theta_counter;
        addrOut = address_counter;
        stateDebug = current_state;
        
        if theta_counter >= thetaMax && address_counter >= rhoMax
            address_counter = fi(0, 0, 16, 0);
            theta_counter = fi(0, 0, 8, 0);
            current_state = CLEAR;
        elseif address_counter >= rhoMax
            address_counter = fi(0, 0, 16, 0);
            theta_counter = fi(theta_counter + 1, 0, 8, 0);
        else
            address_counter = fi(address_counter + 1, 0, 16, 0);
        end
        
    case CLEAR
        sofOut = false;
        eofOut = false; 
        validOut = false;
        modeOut = true;
        voteOut = false;
        clearOut = true;
        phaseOut = false;
        thetaOut = theta_counter;
        addrOut = address_counter;
        stateDebug = current_state;
        
        if address_counter >= rhoMax
            address_counter = fi(0, 0, 16, 0);
            current_state = IDLE;
        else
            address_counter = fi(address_counter + 1, 0, 16, 0);
        end
        
    otherwise
        sofOut = false;
        eofOut = false; 
        validOut = false;
        modeOut = false;
        voteOut = false;
        clearOut = false;
        phaseOut = false;
        thetaOut = theta_counter;
        addrOut = address_counter;
        stateDebug = current_state;
        
        current_state = IDLE;
        
end
